simulink model "D53_LKAS"  (R2018b)
settings: Solver=ode3  StartTime=0.0  StopTime=10  FixedStep=0.01  RelTol=1e-3  EnableMultiTasking=on
model workspace (MAT data in the model file):
  MCOS : class17 (value not decoded)
  MCOS : class17 (value not decoded)
  MCOS : class17 (value not decoded)
  MCOS : class17 (value not decoded)
  MCOS : class17 (value not decoded)
  MCOS : class17 (value not decoded)
  MCOS : class17 (value not decoded)
  MCOS : class17 (value not decoded)
  MCOS : class17 (value not decoded)
  MCOS : class17 (value not decoded)
  MCOS : class17 (value not decoded)
  MCOS : class17 (value not decoded)
  MCOS : class17 (value not decoded)
  MCOS : class17 (value not decoded)
  MCOS : class17 (value not decoded)
  MCOS : class17 (value not decoded)
  MCOS : class17 (value not decoded)
  MCOS : class17 (value not decoded)
  MCOS : class17 (value not decoded)
  MCOS : class17 (value not decoded)
  MCOS : class17 (value not decoded)
  MCOS : class17 (value not decoded)
  MCOS : class17 (value not decoded)
  MCOS : class17 (value not decoded)
  MCOS : class17 (value not decoded)
  MCOS : class17 (value not decoded)
  MCOS : class17 (value not decoded)
  MCOS : class17 (value not decoded)
  MCOS : class17 (value not decoded)
  MCOS : class17 (value not decoded)
  MCOS : class17 (value not decoded)
  MCOS : class17 (value not decoded)
  MCOS : class17 (value not decoded)
  MCOS : class17 (value not decoded)
  MCOS : class17 (value not decoded)
  MCOS : class17 (value not decoded)
  MCOS : class17 (value not decoded)
  MCOS : class17 (value not decoded)
  MCOS : class17 (value not decoded)
  MCOS : class17 (value not decoded)
  MCOS : class17 (value not decoded)
  MCOS : class17 (value not decoded)
  MCOS : class17 (value not decoded)
  MCOS : class17 (value not decoded)
  MCOS : class17 (value not decoded)
  MCOS : class17 (value not decoded)
  MCOS : class17 (value not decoded)
  MCOS : class17 (value not decoded)
  MCOS : class17 (value not decoded)
  MCOS : class17 (value not decoded)
  MCOS : class17 (value not decoded)
  MCOS : class17 (value not decoded)
  MCOS : class17 (value not decoded)
  MCOS : class17 (value not decoded)
  MCOS : class17 (value not decoded)
  MCOS : class17 (value not decoded)
  MCOS : class17 (value not decoded)
  MCOS : class17 (value not decoded)
  MCOS : class17 (value not decoded)
  MCOS : class17 (value not decoded)
  MCOS : class17 (value not decoded)
  MCOS : class17 (value not decoded)
  MCOS : class17 (value not decoded)
  MCOS : class17 (value not decoded)
  MCOS : class17 (value not decoded)
  MCOS : class17 (value not decoded)
  MCOS : class17 (value not decoded)
  MCOS : class17 (value not decoded)
  MCOS : class17 (value not decoded)
  MCOS : class17 (value not decoded)
  MCOS : class17 (value not decoded)
  MCOS : class17 (value not decoded)
  MCOS : class17 (value not decoded)
  MCOS : class17 (value not decoded)
  MCOS : class17 (value not decoded)
  MCOS : class17 (value not decoded)
  MCOS : class17 (value not decoded)
  MCOS : class17 (value not decoded)
  MCOS : class17 (value not decoded)
  MCOS : class17 (value not decoded)
  MCOS : class17 (value not decoded)
  MCOS : class17 (value not decoded)
  MCOS : class17 (value not decoded)
  MCOS : class17 (value not decoded)
  MCOS : class17 (value not decoded)
  MCOS : class17 (value not decoded)
  MCOS : class17 (value not decoded)
  MCOS : class17 (value not decoded)
  MCOS : class17 (value not decoded)
values from neighbouring files (symbols this model uses):
  C = who    [Data_Process.m]
undefined symbols (not defined in the file or in its folder): LKA_CarWidth, LKA_SampleTime, LKA_StrRatio_C, LKA_Veh2CamL_C, LKA_Veh2CamW_C, LKA_WhlBaseL_C, LL_CompSWA_C, LL_CrvtPrvwT_C, LL_DesDvt_C, LL_DvtComp_C, LL_DvtPrvwT_C, LL_DvtSpdDet_vDvtSpdMin_C, LL_HdAgExT_C, LL_HdAgPrvwT_C, LL_LAccMax_C, LL_LAccRMax_C, LL_LDW_EarliestWarnLine_C, LL_LDW_LatestWarnLine_C, LL_LDWS_SUPPRESS_HEADING, LL_LFClb_TFC_DiffCtlBalance, LL_LFClb_TFC_DiffCtrlMaxSWA, LL_LFClb_TFC_DiffCtrlRatio, LL_LFClb_TFC_facmGainLutGain1_C, LL_LFClb_TFC_facmGainLutGain2_C, LL_LFClb_TFC_facmIntegRatio, LL_LFClb_TFC_facmKlat_C, LL_LFClb_TFC_FfCtlRatio_C, LL_LFClb_TFC_phiIntegCtlMaxSWA_C, LL_LFClb_TFC_tiKlatPrvwT_C, LL_LFClb_TFC_vGainLutVehSpdLwr_C, LL_LFClb_TFC_vGainLutVehSpdUpr_C, LL_LKA_EarliestWarnLine_C, LL_LKA_LatestWarnLine_C, LL_LKAExPrcs_ExitC0Dvt, LL_LKAExPrcs_ExitC0Swt, LL_LKAExPrcs_tiExitTime1, LL_LKAExPrcs_tiExitTime2, LL_LKAExPrcs_tiExitTime3, LL_LKAS_OUT_OF_CONTROL_LAT_VEL, LL_LKAS_OUT_OF_CONTROL_TTLC, LL_LKASWASyn_M0, LL_LKASWASyn_M1, LL_LKASWASyn_M2, LL_LKASWASyn_M3K, LL_LKASWASyn_SWAaddMax, LL_LKASWASyn_T2, LL_LKASWASyn_tiTrqSwaRtTime, LL_LKASWASyn_tiTrqSwaTime, LL_LKASWASyn_TrqMax, LL_LKASWASyn_TrqSwaAddSwt, LL_LKASWASyn_TrqSwaRateDiff, LL_LSpdCompT_C, LL_lStpLngth_C, LL_MAX_DELAY_EPSSTAR_TIME, LL_MAX_DRIVER_TORQUE_DISABLE, LL_MAX_DRIVER_TORQUE_ENABLE, LL_MAX_LANE_WIDTH_DISABLE, LL_MAX_LANE_WIDTH_ENABLE, LL_MAX_LAT_ACC_DISABLE, LL_MAX_LAT_ACC_ENABLE ... (+30)
libraries: simulink x134, canmsglib x52, dspstat3 x3, simulink_extras x1
(part 6 of 18)

== system D53_LKAS/SignalBusCreator/bsOriR0Info ==
  Bus Creator21 : BusCreator  Inputs=10
  CAN Pack : canmsglib/CAN Pack  CANdbFile=D:\LKAS\Documents\LKAS-Monitor.dbc  MsgList=Video_Lane_Right_B  MsgName=Video_Lane_Right_B  MsgIDType=Standard (11-bit identifier)  MsgIdentifier=1791  MsgLength=4  SignalInfo=Line_Width_5FF$17$7$2$2$1$0$1.000000e-02$0$0$1.270000e+00$#Me_Line_Changed_5FF$16$1$2$2$1$0$1$0$0$1$#TLC_5FF$8$8$2$2$1$0$1.000000e-02$0$0$2.550000e+00$#View_Range_5FF$0$8$2$2$1$0$5.000000e-01$0$0$1.275000e+02$#  NSignals=4  StartBits=str2num('[int32(17);int32(16);int32(8);int32(0)]')  SignalSizes=str2num('[int32(7);int32(1);int32(8);int32(8)]')  ByteOrders=str2num('[int32(2);int32(2);int32(2);int32(2)]')  DataTypes=str2num('[int32(2);int32(2);int32(2);int32(2)]')  MultiplexTypes=str2num('[int32(1);int32(1);int32(1);int32(1)]')  MultiplexValues=str2num('[double(0);double(0);double(0);double(0)]')  Factors=str2num('[double(1.000000e-02);double(1);double(1.000000e-02);double(5.000000e-01)]')  Offsets=str2num('[double(0);double(0);double(0);double(0)]')  Minimums=str2num('[double(0);double(0);double(0);double(0)]')  Maximums=str2num('[double(1.270000e+00);double(1);double(2.550000e+00);double(1.275000e+02)]')  Remote=off  ApplyMinMax=off  BusOutput=off
      settings: SourceProductName=Simulink Real-Time  SourceProductBaseCode=XP  DataFormat=CANdb specified signals
  CAN Pack1 : canmsglib/CAN Pack  CANdbFile=D:\LKAS\Documents\LKAS-Monitor.dbc  MsgList=Video_Lane_Right_A  MsgName=Video_Lane_Right_A  MsgIDType=Standard (11-bit identifier)  MsgIdentifier=1789  MsgLength=8  SignalInfo=C0_5FD$44$12$2$1$1$0$1.000000e-02$0$-2.048000e+01$2.047000e+01$#C1_5FD$50$10$2$1$1$0$9.765625e-04$0$-3.570000e-01$3.570000e-01$#C2_5FD$24$16$2$1$1$0$1.000000e-06$0$-3.276800e-02$3.276600e-02$#C3_5FD$8$16$2$1$1$0$4.000000e-09$0$-1.310720e-04$1.310680e-04$#Line_Type_5FD$59$3$2$2$1$0$1$0$0$7$#Quality_5FD$62$2$2$2$1$0$1$0$0$3$#  NSignals=6  StartBits=str2num('[int32(44);int32(50);int32(24);int32(8);int32(59);int32(62)]')  SignalSizes=str2num('[int32(12);int32(10);int32(16);int32(16);int32(3);int32(2)]')  ByteOrders=str2num('[int32(2);int32(2);int32(2);int32(2);int32(2);int32(2)]')  DataTypes=str2num('[int32(1);int32(1);int32(1);int32(1);int32(2);int32(2)]')  MultiplexTypes=str2num('[int32(1);int32(1);int32(1);int32(1);int32(1);int32(1)]')  MultiplexValues=str2num('[double(0);double(0);double(0);double(0);double(0);double(0)]')  Factors=str2num('[double(1.000000e-02);double(9.765625e-04);double(1.000000e-06);double(4.000000e-09);double(1);double(1)]')  Offsets=str2num('[double(0);double(0);double(0);double(0);double(0);double(0)]')  Minimums=str2num('[double(-2.048000e+01);double(-3.570000e-01);double(-3.276800e-02);double(-1.310720e-04);double(0);double(0)]')  Maximums=str2num('[double(2.047000e+01);double(3.570000e-01);double(3.276600e-02);double(1.310680e-04);double(7);double(3)]')  Remote=off  ApplyMinMax=off  BusOutput=off
      settings: SourceProductName=Simulink Real-Time  SourceProductBaseCode=XP  DataFormat=CANdb specified signals
  CAN Pack2 : canmsglib/CAN Pack  CANdbFile=D:\LKAS\Documents\D53-PSA1CAN.dbc  MsgList=ADAS_44B_PSA1  MsgName=ADAS_44B_PSA1  MsgIDType=Standard (11-bit identifier)  MsgIdentifier=1099  MsgLength=8  SignalInfo=C0_coefficient44B$44$12$2$1$1$0$1.000000e-02$0$-2.048000e+01$2.047000e+01$#C1_coefficient44B$50$10$2$1$1$0$9.800000e-04$0$-3.570000e-01$3.570000e-01$#C2_coefficient44B$24$16$2$1$1$0$1.000000e-06$0$-3.276800e-02$3.276600e-02$#C3_coefficient44B$8$16$2$1$1$0$4.000000e-09$0$-1.310000e-04$1.310700e-04$#Detected_line_type44B$59$3$2$2$1$0$1$0$0$7$#Message_counter44B$48$2$2$2$1$0$1$0$0$3$#Quality_of_the_detected_line44B$62$2$2$2$1$0$1$0$0$3$#  NSignals=7  StartBits=str2num('[int32(44);int32(50);int32(24);int32(8);int32(59);int32(48);int32(62)]')  SignalSizes=str2num('[int32(12);int32(10);int32(16);int32(16);int32(3);int32(2);int32(2)]')  ByteOrders=str2num('[int32(2);int32(2);int32(2);int32(2);int32(2);int32(2);int32(2)]')  DataTypes=str2num('[int32(1);int32(1);int32(1);int32(1);int32(2);int32(2);int32(2)]')  MultiplexTypes=str2num('[int32(1);int32(1);int32(1);int32(1);int32(1);int32(1);int32(1)]')  MultiplexValues=str2num('[double(0);double(0);double(0);double(0);double(0);double(0);double(0)]')  Factors=str2num('[double(1.000000e-02);double(9.800000e-04);double(1.000000e-06);double(4.000000e-09);double(1);double(1);double(1)]')  Offsets=str2num('[double(0);double(0);double(0);double(0);double(0);double(0);double(0)]')  Minimums=str2num('[double(-2.048000e+01);double(-3.570000e-01);double(-3.276800e-02);double(-1.310000e-04);double(0);double(0);double(0)]')  Maximums=str2num('[double(2.047000e+01);double(3.570000e-01);double(3.276600e-02);double(1.310700e-04);double(7);double(3);double(3)]')  Remote=off  ApplyMinMax=off  BusOutput=off
      settings: SourceProductName=Simulink Real-Time  SourceProductBaseCode=XP  DataFormat=CANdb specified signals
  CAN Receive (CANRX) : S-Function  FunctionName=CAN_Rec_P  Parameters=uint8(Module-1),uint32(ID),uint8(Frameformat-1),uint8(Newflag),uint8(FIFO),double(sampletime)  SFunctionDeploymentMode=off  EnableBusSupport=off  mask(CAN_receive){Module=CAN_2, ID=1533, Frameformat=Standard (11-bit identifier), Newflag=on, FIFO=off, sampletime=0.05}
      mask prompts: Module "CAN Port:"; ID "CAN Frame ID:"; Frameformat "CAN Frame Format:"; FIFO "Overflow flag"
      mask init:
      | maskdisplay = canrecicon(Module,ID,Frameformat,Newflag,FIFO);
      | set_param(gcb, 'MaskDisplay', maskdisplay);
      mask TypeOptions Module: CAN_0 | CAN_1 | CAN_2 | CAN_3
      mask TypeOptions Frameformat: Standard (11-bit identifier) | Extended (29-bit identifier)
      mask Display: color('blue');text(0.98,0.9,'MPC5675K','horizontalAlignment','right');color('black');text(0.5,0.6,'FlexCAN_2 Receive','horizontalAlignment','center');text(0.5,0.35,'Standard ID:1533','horizontalAlignment','center');port_label('output',1,'New_Flag');port_label('output',2,'CAN_Msg');
  CAN Receive (CANRX)1 : S-Function  FunctionName=CAN_Rec_P  Parameters=uint8(Module-1),uint32(ID),uint8(Frameformat-1),uint8(Newflag),uint8(FIFO),double(sampletime)  SFunctionDeploymentMode=off  EnableBusSupport=off  mask(CAN_receive){Module=CAN_2, ID=1535, Frameformat=Standard (11-bit identifier), Newflag=on, FIFO=off, sampletime=0.05}
      mask prompts: Module "CAN Port:"; ID "CAN Frame ID:"; Frameformat "CAN Frame Format:"; FIFO "Overflow flag"
      mask init:
      | maskdisplay = canrecicon(Module,ID,Frameformat,Newflag,FIFO);
      | set_param(gcb, 'MaskDisplay', maskdisplay);
      mask TypeOptions Module: CAN_0 | CAN_1 | CAN_2 | CAN_3
      mask TypeOptions Frameformat: Standard (11-bit identifier) | Extended (29-bit identifier)
      mask Display: color('blue');text(0.98,0.9,'MPC5675K','horizontalAlignment','right');color('black');text(0.5,0.6,'FlexCAN_2 Receive','horizontalAlignment','center');text(0.5,0.35,'Standard ID:1535','horizontalAlignment','center');port_label('output',1,'New_Flag');port_label('output',2,'CAN_Msg');
  CAN Send1 : S-Function  FunctionName=CAN_Send_P  Parameters=uint8(CAN_Port-1),uint8(CAN_Priority-1),uint8(S_overflow_flag),uint8(S_timestamp),double(sampletime)  SFunctionDeploymentMode=off  EnableBusSupport=off  mask{CAN_Port=CAN_1, CAN_Priority=3, S_overflow_flag=off, S_timestamp=off, sampletime=0.05}
      mask prompts: CAN_Port "CAN Port:"; CAN_Priority "Priority:"; S_overflow_flag "Send overflow flag"; S_timestamp "Send time stamp"
      mask init:
      | maskdisplay = cansendicon(CAN_Port,CAN_Priority,S_overflow_flag,S_timestamp);
      | set_param(gcb, 'MaskDisplay', maskdisplay);
      mask TypeOptions CAN_Port: CAN_0 | CAN_1 | CAN_2 | CAN_3
      mask TypeOptions CAN_Priority: 0 | 1 | 2 | 3 | 4 | 5 | 6 | 7
      mask Display: color('blue');text(0.98,0.9,'MPC5675K','horizontalAlignment','right');color('black');text(0.5,0.6,'FlexCAN_1 Send','horizontalAlignment','center');text(0.5,0.35,'Priority:3','horizontalAlignment','center');port_label('input',1,'CAN_Msg');
  CAN Send2 : S-Function  FunctionName=CAN_Send_P  Parameters=uint8(CAN_Port-1),uint8(CAN_Priority-1),uint8(S_overflow_flag),uint8(S_timestamp),double(sampletime)  SFunctionDeploymentMode=off  EnableBusSupport=off  mask{CAN_Port=CAN_0, CAN_Priority=3, S_overflow_flag=off, S_timestamp=off, sampletime=0.05}
      mask prompts: CAN_Port "CAN Port:"; CAN_Priority "Priority:"; S_overflow_flag "Send overflow flag"; S_timestamp "Send time stamp"
      mask init:
      | maskdisplay = cansendicon(CAN_Port,CAN_Priority,S_overflow_flag,S_timestamp);
      | set_param(gcb, 'MaskDisplay', maskdisplay);
      mask TypeOptions CAN_Port: CAN_0 | CAN_1 | CAN_2 | CAN_3
      mask TypeOptions CAN_Priority: 0 | 1 | 2 | 3 | 4 | 5 | 6 | 7
      mask Display: color('blue');text(0.98,0.9,'MPC5675K','horizontalAlignment','right');color('black');text(0.5,0.6,'FlexCAN_0 Send','horizontalAlignment','center');text(0.5,0.35,'Priority:3','horizontalAlignment','center');port_label('input',1,'CAN_Msg');
  CAN Send3 : S-Function  FunctionName=CAN_Send_P  Parameters=uint8(CAN_Port-1),uint8(CAN_Priority-1),uint8(S_overflow_flag),uint8(S_timestamp),double(sampletime)  SFunctionDeploymentMode=off  EnableBusSupport=off  mask{CAN_Port=CAN_0, CAN_Priority=3, S_overflow_flag=off, S_timestamp=off, sampletime=0.05}
      mask prompts: CAN_Port "CAN Port:"; CAN_Priority "Priority:"; S_overflow_flag "Send overflow flag"; S_timestamp "Send time stamp"
      mask init:
      | maskdisplay = cansendicon(CAN_Port,CAN_Priority,S_overflow_flag,S_timestamp);
      | set_param(gcb, 'MaskDisplay', maskdisplay);
      mask TypeOptions CAN_Port: CAN_0 | CAN_1 | CAN_2 | CAN_3
      mask TypeOptions CAN_Priority: 0 | 1 | 2 | 3 | 4 | 5 | 6 | 7
      mask Display: color('blue');text(0.98,0.9,'MPC5675K','horizontalAlignment','right');color('black');text(0.5,0.6,'FlexCAN_0 Send','horizontalAlignment','center');text(0.5,0.35,'Priority:3','horizontalAlignment','center');port_label('input',1,'CAN_Msg');
  CAN Unpack1 : canmsglib/CAN Unpack  CANdbFile=D:\Work\02_LKA\LKAS\Documents\D53-SensorCAN.dbc  MsgList=Video_Lane_Right_B  MsgName=Video_Lane_Right_B  MsgIDType=Standard (11-bit identifier)  MsgIdentifier=1535  MsgLength=4  SignalInfo=Line_Width_5FF$17$7$2$2$1$0$1.000000e-02$0$0$1.270000e+00$#Me_Line_Changed_5FF$16$1$2$2$1$0$1$0$0$1$#TLC_5FF$8$8$2$2$1$0$1.000000e-02$0$0$2.550000e+00$#View_Range_5FF$0$8$2$2$1$0$5.000000e-01$0$0$1.275000e+02$#  NSignals=4  IDPort=off  TimestampPort=off  ErrorPort=off  RemotePort=off  LengthPort=off  StatusPort=off  StartBits=str2num('[int32(17);int32(16);int32(8);int32(0)]')  SignalSizes=str2num('[int32(7);int32(1);int32(8);int32(8)]')  ByteOrders=str2num('[int32(2);int32(2);int32(2);int32(2)]')  DataTypes=str2num('[int32(2);int32(2);int32(2);int32(2)]')  MultiplexTypes=str2num('[int32(1);int32(1);int32(1);int32(1)]')  MultiplexValues=str2num('[double(0);double(0);double(0);double(0)]')  Factors=str2num('[double(1.000000e-02);double(1);double(1.000000e-02);double(5.000000e-01)]')  Offsets=str2num('[double(0);double(0);double(0);double(0)]')  Minimums=str2num('[double(0);double(0);double(0);double(0)]')  Maximums=str2num('[double(1.270000e+00);double(1);double(2.550000e+00);double(1.275000e+02)]')  ApplyMinMax=off
      settings: SourceProductName=Simulink Real-Time  SourceProductBaseCode=XP  DataFormat=CANdb specified signals
  CAN Unpack14 : canmsglib/CAN Unpack  CANdbFile=D:\Work\02_LKA\LKAS\Documents\D53-SensorCAN.dbc  MsgList=Video_Lane_Right_A  MsgName=Video_Lane_Right_A  MsgIDType=Standard (11-bit identifier)  MsgIdentifier=1533  MsgLength=8  SignalInfo=C0_5FD$44$12$2$1$1$0$1.000000e-02$0$-2.048000e+01$2.047000e+01$#C1_5FD$50$10$2$1$1$0$9.765625e-04$0$-3.570000e-01$3.570000e-01$#C2_5FD$24$16$2$1$1$0$1.000000e-06$0$-3.276800e-02$3.276600e-02$#C3_5FD$8$16$2$1$1$0$4.000000e-09$0$-1.310720e-04$1.310680e-04$#Line_Type_5FD$59$3$2$2$1$0$1$0$0$7$#Quality_5FD$62$2$2$2$1$0$1$0$0$3$#  NSignals=6  IDPort=off  TimestampPort=off  ErrorPort=off  RemotePort=off  LengthPort=off  StatusPort=off  StartBits=str2num('[int32(44);int32(50);int32(24);int32(8);int32(59);int32(62)]')  SignalSizes=str2num('[int32(12);int32(10);int32(16);int32(16);int32(3);int32(2)]')  ByteOrders=str2num('[int32(2);int32(2);int32(2);int32(2);int32(2);int32(2)]')  DataTypes=str2num('[int32(1);int32(1);int32(1);int32(1);int32(2);int32(2)]')  MultiplexTypes=str2num('[int32(1);int32(1);int32(1);int32(1);int32(1);int32(1)]')  MultiplexValues=str2num('[double(0);double(0);double(0);double(0);double(0);double(0)]')  Factors=str2num('[double(1.000000e-02);double(9.765625e-04);double(1.000000e-06);double(4.000000e-09);double(1);double(1)]')  Offsets=str2num('[double(0);double(0);double(0);double(0);double(0);double(0)]')  Minimums=str2num('[double(-2.048000e+01);double(-3.570000e-01);double(-3.276800e-02);double(-1.310720e-04);double(0);double(0)]')  Maximums=str2num('[double(2.047000e+01);double(3.570000e-01);double(3.276600e-02);double(1.310680e-04);double(7);double(3)]')  ApplyMinMax=off
      settings: SourceProductName=Simulink Real-Time  SourceProductBaseCode=XP  DataFormat=CANdb specified signals
  Data Type Conversion{1..4,6..7,10} (7 alike) : DataTypeConversion  OutDataTypeStr=single
  Data Type Conversion5 : DataTypeConversion  OutDataTypeStr=uint8
  Data Type Conversion8 : DataTypeConversion  OutDataTypeStr=uint8
  Data Type Conversion9 : DataTypeConversion  OutDataTypeStr=uint8
  Ground : Ground
  Rate Transition{1..10} (10 alike) : RateTransition  Deterministic=off  OutPortSampleTime=0.01
  Rate Transition{11..27} (17 alike) : RateTransition  Deterministic=off  OutPortSampleTime=0.05
  bsOriR0Info : Outport
  wires:
  Data Type Conversion4/1 -> Rate Transition11/1, Rate Transition18/1, Bus Creator21/4  "O_R0_C0"
  CAN Unpack1/4 -> Rate Transition1/1
  Data Type Conversion1/1 -> Rate Transition12/1, Rate Transition19/1, Bus Creator21/3  "O_R0_C1"
  Data Type Conversion7/1 -> Rate Transition24/1, Bus Creator21/9  "O_R0_W"
  Data Type Conversion10/1 -> Rate Transition26/1, Bus Creator21/8  "O_R0_TLC"
  CAN Unpack1/2 -> Rate Transition3/1
  Data Type Conversion9/1 -> Rate Transition25/1, Bus Creator21/10  "O_R0_LC"
  Data Type Conversion6/1 -> Rate Transition27/1, Bus Creator21/7  "O_R0_VR"
  CAN Unpack14/1 -> Rate Transition10/1
  Data Type Conversion2/1 -> Rate Transition20/1, Rate Transition13/1, Bus Creator21/2  "O_R0_C2"
  CAN Unpack14/3 -> Rate Transition8/1
  CAN Unpack1/3 -> Rate Transition2/1
  Data Type Conversion8/1 -> Rate Transition22/1, Rate Transition15/1, Bus Creator21/6  "O_R0_Type"
  Data Type Conversion3/1 -> Rate Transition21/1, Rate Transition14/1, Bus Creator21/1  "O_R0_C3"
  CAN Unpack14/6 -> Rate Transition5/1
  CAN Unpack14/2 -> Rate Transition9/1
  CAN Unpack14/4 -> Rate Transition7/1
  CAN Unpack14/5 -> Rate Transition6/1
  Data Type Conversion5/1 -> Rate Transition23/1, Rate Transition16/1, Bus Creator21/5  "O_R0_Q"
  CAN Unpack1/1 -> Rate Transition4/1
  Bus Creator21/1 -> bsOriR0Info/1  "bsOriR0Info"
  Rate Transition1/1 -> Data Type Conversion6/1
  Rate Transition2/1 -> Data Type Conversion10/1
  Rate Transition3/1 -> Data Type Conversion9/1
  Rate Transition4/1 -> Data Type Conversion7/1
  Rate Transition5/1 -> Data Type Conversion5/1
  Rate Transition6/1 -> Data Type Conversion8/1
  Rate Transition7/1 -> Data Type Conversion3/1
  Rate Transition9/1 -> Data Type Conversion1/1
  Rate Transition8/1 -> Data Type Conversion2/1
  Rate Transition10/1 -> Data Type Conversion4/1
  CAN Pack/1 -> CAN Send3/1
  CAN Pack1/1 -> CAN Send2/1
  Ground/1 -> Rate Transition17/1
  CAN Pack2/1 -> CAN Send1/1
  Rate Transition11/1 -> CAN Pack2/1
  Rate Transition12/1 -> CAN Pack2/2
  Rate Transition13/1 -> CAN Pack2/3
  Rate Transition14/1 -> CAN Pack2/4
  Rate Transition15/1 -> CAN Pack2/5
  Rate Transition16/1 -> CAN Pack2/7
  Rate Transition17/1 -> CAN Pack2/6
  Rate Transition18/1 -> CAN Pack1/1
  Rate Transition19/1 -> CAN Pack1/2
  Rate Transition20/1 -> CAN Pack1/3
  Rate Transition21/1 -> CAN Pack1/4
  Rate Transition22/1 -> CAN Pack1/5
  Rate Transition23/1 -> CAN Pack1/6
  Rate Transition24/1 -> CAN Pack/1
  Rate Transition25/1 -> CAN Pack/2
  Rate Transition26/1 -> CAN Pack/3
  Rate Transition27/1 -> CAN Pack/4
  CAN Receive (CANRX)/2 -> CAN Unpack14/1
  CAN Receive (CANRX)1/2 -> CAN Unpack1/1

== system D53_LKAS/SignalBusCreator/bsOriR1Info ==
  Bus Creator22 : BusCreator  Inputs=10
  CAN Receive (CANRX) : S-Function  FunctionName=CAN_Rec_P  Parameters=uint8(Module-1),uint32(ID),uint8(Frameformat-1),uint8(Newflag),uint8(FIFO),double(sampletime)  SFunctionDeploymentMode=off  EnableBusSupport=off  mask(CAN_receive){Module=CAN_2, ID=1534, Frameformat=Standard (11-bit identifier), Newflag=on, FIFO=off, sampletime=0.05}
      mask prompts: Module "CAN Port:"; ID "CAN Frame ID:"; Frameformat "CAN Frame Format:"; FIFO "Overflow flag"
      mask init:
      | maskdisplay = canrecicon(Module,ID,Frameformat,Newflag,FIFO);
      | set_param(gcb, 'MaskDisplay', maskdisplay);
      mask TypeOptions Module: CAN_0 | CAN_1 | CAN_2 | CAN_3
      mask TypeOptions Frameformat: Standard (11-bit identifier) | Extended (29-bit identifier)
      mask Display: color('blue');text(0.98,0.9,'MPC5675K','horizontalAlignment','right');color('black');text(0.5,0.6,'FlexCAN_2 Receive','horizontalAlignment','center');text(0.5,0.35,'Standard ID:1534','horizontalAlignment','center');port_label('output',1,'New_Flag');port_label('output',2,'CAN_Msg');
  CAN Receive (CANRX)1 : S-Function  FunctionName=CAN_Rec_P  Parameters=uint8(Module-1),uint32(ID),uint8(Frameformat-1),uint8(Newflag),uint8(FIFO),double(sampletime)  SFunctionDeploymentMode=off  EnableBusSupport=off  mask(CAN_receive){Module=CAN_2, ID=1524, Frameformat=Standard (11-bit identifier), Newflag=on, FIFO=off, sampletime=0.05}
      mask prompts: Module "CAN Port:"; ID "CAN Frame ID:"; Frameformat "CAN Frame Format:"; FIFO "Overflow flag"
      mask init:
      | maskdisplay = canrecicon(Module,ID,Frameformat,Newflag,FIFO);
      | set_param(gcb, 'MaskDisplay', maskdisplay);
      mask TypeOptions Module: CAN_0 | CAN_1 | CAN_2 | CAN_3
      mask TypeOptions Frameformat: Standard (11-bit identifier) | Extended (29-bit identifier)
      mask Display: color('blue');text(0.98,0.9,'MPC5675K','horizontalAlignment','right');color('black');text(0.5,0.6,'FlexCAN_2 Receive','horizontalAlignment','center');text(0.5,0.35,'Standard ID:1524','horizontalAlignment','center');port_label('output',1,'New_Flag');port_label('output',2,'CAN_Msg');
  CAN Unpack1 : canmsglib/CAN Unpack  CANdbFile=D:\Work\02_LKA\LKAS\Documents\D53-SensorCAN.dbc  MsgList=Video_Lane_Next_Right_B  MsgName=Video_Lane_Next_Right_B  MsgIDType=Standard (11-bit identifier)  MsgIdentifier=1524  MsgLength=4  SignalInfo=Line_Width_5F4$17$7$2$2$1$0$1.000000e-02$0$0$1.270000e+00$#Me_Line_Changed_5F4$16$1$2$2$1$0$1$0$0$1$#TLC_5F4$8$8$2$2$1$0$1.000000e-02$0$0$2.550000e+00$#View_Range_5F4$0$8$2$2$1$0$5.000000e-01$0$0$1.275000e+02$#  NSignals=4  IDPort=off  TimestampPort=off  ErrorPort=off  RemotePort=off  LengthPort=off  StatusPort=off  StartBits=str2num('[int32(17);int32(16);int32(8);int32(0)]')  SignalSizes=str2num('[int32(7);int32(1);int32(8);int32(8)]')  ByteOrders=str2num('[int32(2);int32(2);int32(2);int32(2)]')  DataTypes=str2num('[int32(2);int32(2);int32(2);int32(2)]')  MultiplexTypes=str2num('[int32(1);int32(1);int32(1);int32(1)]')  MultiplexValues=str2num('[double(0);double(0);double(0);double(0)]')  Factors=str2num('[double(1.000000e-02);double(1);double(1.000000e-02);double(5.000000e-01)]')  Offsets=str2num('[double(0);double(0);double(0);double(0)]')  Minimums=str2num('[double(0);double(0);double(0);double(0)]')  Maximums=str2num('[double(1.270000e+00);double(1);double(2.550000e+00);double(1.275000e+02)]')  ApplyMinMax=off
      settings: SourceProductName=Simulink Real-Time  SourceProductBaseCode=XP  DataFormat=CANdb specified signals
  CAN Unpack13 : canmsglib/CAN Unpack  CANdbFile=D:\Work\02_LKA\LKAS\Documents\D53-SensorCAN.dbc  MsgList=Video_Lane_Next_Right_A  MsgName=Video_Lane_Next_Right_A  MsgIDType=Standard (11-bit identifier)  MsgIdentifier=1534  MsgLength=8  SignalInfo=C0_5FE$44$12$2$1$1$0$1.000000e-02$0$-2.048000e+01$2.047000e+01$#C1_5FE$50$10$2$1$1$0$9.765625e-04$0$-3.570000e-01$3.570000e-01$#C2_5FE$24$16$2$1$1$0$1.000000e-06$0$-3.276800e-02$3.276600e-02$#C3_5FE$8$16$2$1$1$0$4.000000e-09$0$-1.310720e-04$1.310680e-04$#Line_Type_5FE$59$3$2$2$1$0$1$0$0$7$#Quality_5FE$62$2$2$2$1$0$1$0$0$3$#  NSignals=6  IDPort=off  TimestampPort=off  ErrorPort=off  RemotePort=off  LengthPort=off  StatusPort=off  StartBits=str2num('[int32(44);int32(50);int32(24);int32(8);int32(59);int32(62)]')  SignalSizes=str2num('[int32(12);int32(10);int32(16);int32(16);int32(3);int32(2)]')  ByteOrders=str2num('[int32(2);int32(2);int32(2);int32(2);int32(2);int32(2)]')  DataTypes=str2num('[int32(1);int32(1);int32(1);int32(1);int32(2);int32(2)]')  MultiplexTypes=str2num('[int32(1);int32(1);int32(1);int32(1);int32(1);int32(1)]')  MultiplexValues=str2num('[double(0);double(0);double(0);double(0);double(0);double(0)]')  Factors=str2num('[double(1.000000e-02);double(9.765625e-04);double(1.000000e-06);double(4.000000e-09);double(1);double(1)]')  Offsets=str2num('[double(0);double(0);double(0);double(0);double(0);double(0)]')  Minimums=str2num('[double(-2.048000e+01);double(-3.570000e-01);double(-3.276800e-02);double(-1.310720e-04);double(0);double(0)]')  Maximums=str2num('[double(2.047000e+01);double(3.570000e-01);double(3.276600e-02);double(1.310680e-04);double(7);double(3)]')  ApplyMinMax=off
      settings: SourceProductName=Simulink Real-Time  SourceProductBaseCode=XP  DataFormat=CANdb specified signals
  Data Type Conversion{,6..8,10..11,14} (7 alike) : DataTypeConversion  OutDataTypeStr=single
  Data Type Conversion12 : DataTypeConversion  OutDataTypeStr=uint8
  Data Type Conversion13 : DataTypeConversion  OutDataTypeStr=uint8
  Data Type Conversion9 : DataTypeConversion  OutDataTypeStr=uint8
  Rate Transition{1..10} (10 alike) : RateTransition  Deterministic=off  OutPortSampleTime=0.01
  bsOriR1Info : Outport
  wires:
  Data Type Conversion6/1 -> Bus Creator22/3  "O_R1_C1"
  Data Type Conversion11/1 -> Bus Creator22/9  "O_R1_W"
  Data Type Conversion14/1 -> Bus Creator22/8  "O_R1_TLC"
  Data Type Conversion/1 -> Bus Creator22/4  "O_R1_C0"
  Data Type Conversion7/1 -> Bus Creator22/2  "O_R1_C2"
  Data Type Conversion9/1 -> Bus Creator22/5  "O_R1_Q"
  Data Type Conversion13/1 -> Bus Creator22/10  "O_R1_LC"
  Data Type Conversion8/1 -> Bus Creator22/1  "O_R1_C3"
  CAN Unpack13/2 -> Rate Transition2/1
  CAN Unpack13/3 -> Rate Transition3/1
  Data Type Conversion12/1 -> Bus Creator22/6  "O_R1_Type"
  Data Type Conversion10/1 -> Bus Creator22/7  "O_R1_VR"
  CAN Unpack13/1 -> Rate Transition1/1
  CAN Unpack1/4 -> Rate Transition10/1
  CAN Unpack1/3 -> Rate Transition9/1
  CAN Unpack13/5 -> Rate Transition5/1
  CAN Unpack13/6 -> Rate Transition6/1
  CAN Unpack1/2 -> Rate Transition8/1
  CAN Unpack1/1 -> Rate Transition7/1
  CAN Unpack13/4 -> Rate Transition4/1
  Bus Creator22/1 -> bsOriR1Info/1  "bsOriR1Info"
  Rate Transition1/1 -> Data Type Conversion/1
  Rate Transition2/1 -> Data Type Conversion6/1
  Rate Transition3/1 -> Data Type Conversion7/1
  Rate Transition4/1 -> Data Type Conversion8/1
  Rate Transition5/1 -> Data Type Conversion12/1
  Rate Transition6/1 -> Data Type Conversion9/1
  Rate Transition7/1 -> Data Type Conversion11/1
  Rate Transition8/1 -> Data Type Conversion13/1
  Rate Transition9/1 -> Data Type Conversion14/1
  Rate Transition10/1 -> Data Type Conversion10/1
  CAN Receive (CANRX)/2 -> CAN Unpack13/1
  CAN Receive (CANRX)1/2 -> CAN Unpack1/1

== system D53_LKAS/SignalBusCreator/bsPTState ==
  Bus Creator4 : BusCreator  Inputs=2
  CAN Pack : canmsglib/CAN Pack  CANdbFile=D:\LKAS\Documents\LKAS-Monitor.dbc  MsgList=GW_349_PSA1  MsgName=GW_349_PSA1  MsgIDType=Standard (11-bit identifier)  MsgIdentifier=840  MsgLength=8  SignalInfo=TCU_Gear_lever_position$24$4$2$2$1$0$1$0$-Inf$Inf$#  NSignals=1  StartBits=str2num('[int32(24)]')  SignalSizes=str2num('[int32(4)]')  ByteOrders=str2num('[int32(2)]')  DataTypes=str2num('[int32(2)]')  MultiplexTypes=str2num('[int32(1)]')  MultiplexValues=str2num('[double(0)]')  Factors=str2num('[double(1)]')  Offsets=str2num('[double(0)]')  Minimums=str2num('[double(-Inf)]')  Maximums=str2num('[double(Inf)]')  Remote=off  ApplyMinMax=off  BusOutput=off
      settings: SourceProductName=Simulink Real-Time  SourceProductBaseCode=XP  DataFormat=CANdb specified signals
  CAN Send1 : S-Function  FunctionName=CAN_Send_P  Parameters=uint8(CAN_Port-1),uint8(CAN_Priority-1),uint8(S_overflow_flag),uint8(S_timestamp),double(sampletime)  SFunctionDeploymentMode=off  EnableBusSupport=off  mask{CAN_Port=CAN_0, CAN_Priority=3, S_overflow_flag=off, S_timestamp=off, sampletime=0.1}
      mask prompts: CAN_Port "CAN Port:"; CAN_Priority "Priority:"; S_overflow_flag "Send overflow flag"; S_timestamp "Send time stamp"
      mask init:
      | maskdisplay = cansendicon(CAN_Port,CAN_Priority,S_overflow_flag,S_timestamp);
      | set_param(gcb, 'MaskDisplay', maskdisplay);
      mask TypeOptions CAN_Port: CAN_0 | CAN_1 | CAN_2 | CAN_3
      mask TypeOptions CAN_Priority: 0 | 1 | 2 | 3 | 4 | 5 | 6 | 7
      mask Display: color('blue');text(0.98,0.9,'MPC5675K','horizontalAlignment','right');color('black');text(0.5,0.6,'FlexCAN_0 Send','horizontalAlignment','center');text(0.5,0.35,'Priority:3','horizontalAlignment','center');port_label('input',1,'CAN_Msg');
  CAN Unpack1 : canmsglib/CAN Unpack  CANdbFile=D:\Work\02_LKA\LKAS\Documents\D53-PSA1CAN.dbc  MsgList=GW_228_PSA1  MsgName=GW_228_PSA1  MsgIDType=Standard (11-bit identifier)  MsgIdentifier=552  MsgLength=8  SignalInfo=EMS_Acceleration_pedal_position$16$8$2$2$1$0$5.000000e-01$0$0$100$#  NSignals=1  IDPort=off  TimestampPort=off  ErrorPort=off  RemotePort=off  LengthPort=off  StatusPort=off  StartBits=str2num('[int32(16)]')  SignalSizes=str2num('[int32(8)]')  ByteOrders=str2num('[int32(2)]')  DataTypes=str2num('[int32(2)]')  MultiplexTypes=str2num('[int32(1)]')  MultiplexValues=str2num('[double(0)]')  Factors=str2num('[double(5.000000e-01)]')  Offsets=str2num('[double(0)]')  Minimums=str2num('[double(0)]')  Maximums=str2num('[double(100)]')  ApplyMinMax=off
      settings: SourceProductName=Simulink Real-Time  SourceProductBaseCode=XP  DataFormat=CANdb specified signals
  CAN Unpack6 : canmsglib/CAN Unpack  CANdbFile=D:\Work\02_LKA\LKAS\Documents\D53-PSA1CAN.dbc  MsgList=GW_349_PSA1  MsgName=GW_349_PSA1  MsgIDType=Standard (11-bit identifier)  MsgIdentifier=841  MsgLength=8  SignalInfo=BV_dynamic_frame_checksum$52$4$2$2$1$0$1$0$-Inf$Inf$#TCU_AGB_Target_position$28$4$2$2$1$0$1$0$-Inf$Inf$#TCU_Gear_lever_position$24$4$2$2$1$0$1$0$-Inf$Inf$#bits_Compute_for_Gear_Box$48$4$2$2$1$0$1$0$0$15$#  NSignals=4  IDPort=off  TimestampPort=off  ErrorPort=off  RemotePort=off  LengthPort=off  StatusPort=off  StartBits=str2num('[int32(52);int32(28);int32(24);int32(48)]')  SignalSizes=str2num('[int32(4);int32(4);int32(4);int32(4)]')  ByteOrders=str2num('[int32(2);int32(2);int32(2);int32(2)]')  DataTypes=str2num('[int32(2);int32(2);int32(2);int32(2)]')  MultiplexTypes=str2num('[int32(1);int32(1);int32(1);int32(1)]')  MultiplexValues=str2num('[double(0);double(0);double(0);double(0)]')  Factors=str2num('[double(1);double(1);double(1);double(1)]')  Offsets=str2num('[double(0);double(0);double(0);double(0)]')  Minimums=str2num('[double(-Inf);double(-Inf);double(-Inf);double(0)]')  Maximums=str2num('[double(Inf);double(Inf);double(Inf);double(15)]')  ApplyMinMax=off
      settings: SourceProductName=Simulink Real-Time  SourceProductBaseCode=XP  DataFormat=CANdb specified signals
  CAN_Receive1 : S-Function  FunctionName=CAN_Rec_P  Parameters=uint8(Module-1),uint32(ID),uint8(Frameformat-1),uint8(Newflag),uint8(FIFO),double(sampletime)  SFunctionDeploymentMode=off  EnableBusSupport=off  mask(CAN_receive){Module=CAN_1, ID=552, Frameformat=Standard (11-bit identifier), Newflag=on, FIFO=off, sampletime=0.01}
      mask prompts: Module "CAN Port:"; ID "CAN Frame ID:"; Frameformat "CAN Frame Format:"; FIFO "Overflow flag"
      mask init:
      | maskdisplay = canrecicon(Module,ID,Frameformat,Newflag,FIFO);
      | set_param(gcb, 'MaskDisplay', maskdisplay);
      mask TypeOptions Module: CAN_0 | CAN_1 | CAN_2 | CAN_3
      mask TypeOptions Frameformat: Standard (11-bit identifier) | Extended (29-bit identifier)
      mask Display: color('blue');text(0.98,0.9,'MPC5675K','horizontalAlignment','right');color('black');text(0.5,0.6,'FlexCAN_1 Receive','horizontalAlignment','center');text(0.5,0.35,'Standard ID:552','horizontalAlignment','center');port_label('output',1,'New_Flag');port_label('output',2,'CAN_Msg');
  CAN_Receive6 : S-Function  FunctionName=CAN_Rec_P  Parameters=uint8(Module-1),uint32(ID),uint8(Frameformat-1),uint8(Newflag),uint8(FIFO),double(sampletime)  SFunctionDeploymentMode=off  EnableBusSupport=off  mask(CAN_receive){Module=CAN_1, ID=841, Frameformat=Standard (11-bit identifier), Newflag=on, FIFO=off, sampletime=0.01}
      mask prompts: Module "CAN Port:"; ID "CAN Frame ID:"; Frameformat "CAN Frame Format:"; FIFO "Overflow flag"
      mask init:
      | maskdisplay = canrecicon(Module,ID,Frameformat,Newflag,FIFO);
      | set_param(gcb, 'MaskDisplay', maskdisplay);
      mask TypeOptions Module: CAN_0 | CAN_1 | CAN_2 | CAN_3
      mask TypeOptions Frameformat: Standard (11-bit identifier) | Extended (29-bit identifier)
      mask Display: color('blue');text(0.98,0.9,'MPC5675K','horizontalAlignment','right');color('black');text(0.5,0.6,'FlexCAN_1 Receive','horizontalAlignment','center');text(0.5,0.35,'Standard ID:841','horizontalAlignment','center');port_label('output',1,'New_Flag');port_label('output',2,'CAN_Msg');
  Data Type Conversion1 : DataTypeConversion  OutDataTypeStr=uint8
  Data Type Conversion7 : DataTypeConversion  OutDataTypeStr=uint8
  Rate Transition1 : RateTransition  OutPortSampleTime=0.01
  Rate Transition{2..5} (4 alike) : RateTransition  Deterministic=off  OutPortSampleTime=0.01
  Rate Transition6 : RateTransition  Deterministic=off  OutPortSampleTime=0.1
  Terminator : Terminator
  Terminator1 : Terminator
  Terminator2 : Terminator
  bsPTState : Outport
  wires:
  CAN Unpack6/3 -> Rate Transition3/1
  Bus Creator4/1 -> bsPTState/1  "bsPTState"
  CAN Unpack6/1 -> Rate Transition2/1
  Data Type Conversion7/1 -> Rate Transition6/1, Bus Creator4/2  "TCU_ActualGear"
  CAN Unpack6/4 -> Rate Transition5/1
  CAN Unpack1/1 -> Rate Transition1/1
  Rate Transition1/1 -> Data Type Conversion1/1
  Data Type Conversion1/1 -> Bus Creator4/1  "AccPedal_Pos"
  CAN Unpack6/2 -> Rate Transition4/1
  Rate Transition3/1 -> Data Type Conversion7/1
  CAN Pack/1 -> CAN Send1/1
  Rate Transition2/1 -> Terminator/1
  Rate Transition4/1 -> Terminator2/1
  Rate Transition5/1 -> Terminator1/1
  Rate Transition6/1 -> CAN Pack/1
  CAN_Receive6/2 -> CAN Unpack6/1
  CAN_Receive1/2 -> CAN Unpack1/1

== system D53_LKAS/SignalBusCreator/bsSWAInfo ==
  Bus Creator3 : BusCreator  Inputs=4
  CAN Pack : canmsglib/CAN Pack  CANdbFile=D:\LKAS\Documents\LKAS-Monitor.dbc  MsgList=EPS_305_PSA1  MsgName=EPS_305_PSA1  MsgIDType=Standard (11-bit identifier)  MsgIdentifier=772  MsgLength=7  SignalInfo=Steering_wheel_angle$8$16$2$1$1$0$1.000000e-01$0$-780$780$#Steering_wheel_rotation_speed$16$8$2$2$1$0$4$0$0$1016$#Steering_wheel_sensor_direction$31$1$2$2$1$0$1$0$-Inf$Inf$#  NSignals=3  StartBits=str2num('[int32(8);int32(16);int32(31)]')  SignalSizes=str2num('[int32(16);int32(8);int32(1)]')  ByteOrders=str2num('[int32(2);int32(2);int32(2)]')  DataTypes=str2num('[int32(1);int32(2);int32(2)]')  MultiplexTypes=str2num('[int32(1);int32(1);int32(1)]')  MultiplexValues=str2num('[double(0);double(0);double(0)]')  Factors=str2num('[double(1.000000e-01);double(4);double(1)]')  Offsets=str2num('[double(0);double(0);double(0)]')  Minimums=str2num('[double(-780);double(0);double(-Inf)]')  Maximums=str2num('[double(780);double(1016);double(Inf)]')  Remote=off  ApplyMinMax=off  BusOutput=off
      settings: SourceProductName=Simulink Real-Time  SourceProductBaseCode=XP  DataFormat=CANdb specified signals
  CAN Recv (CANRx]) : S-Function  FunctionName=CAN_Rec_P  Parameters=uint8(Module-1),uint32(ID),uint8(Frameformat-1),uint8(Newflag),uint8(FIFO),double(sampletime)  SFunctionDeploymentMode=off  EnableBusSupport=off  mask(CAN_receive){Module=CAN_1, ID=773, Frameformat=Standard (11-bit identifier), Newflag=on, FIFO=off, sampletime=0.01}
      mask prompts: Module "CAN Port:"; ID "CAN Frame ID:"; Frameformat "CAN Frame Format:"; FIFO "Overflow flag"
      mask init:
      | maskdisplay = canrecicon(Module,ID,Frameformat,Newflag,FIFO);
      | set_param(gcb, 'MaskDisplay', maskdisplay);
      mask TypeOptions Module: CAN_0 | CAN_1 | CAN_2 | CAN_3
      mask TypeOptions Frameformat: Standard (11-bit identifier) | Extended (29-bit identifier)
      mask Display: color('blue');text(0.98,0.9,'MPC5675K','horizontalAlignment','right');color('black');text(0.5,0.6,'FlexCAN_1 Receive','horizontalAlignment','center');text(0.5,0.35,'Standard ID:773','horizontalAlignment','center');port_label('output',1,'New_Flag');port_label('output',2,'CAN_Msg');
  CAN Send2 : S-Function  FunctionName=CAN_Send_P  Parameters=uint8(CAN_Port-1),uint8(CAN_Priority-1),uint8(S_overflow_flag),uint8(S_timestamp),double(sampletime)  SFunctionDeploymentMode=off  EnableBusSupport=off  mask{CAN_Port=CAN_0, CAN_Priority=3, S_overflow_flag=off, S_timestamp=off, sampletime=0.1}
      mask prompts: CAN_Port "CAN Port:"; CAN_Priority "Priority:"; S_overflow_flag "Send overflow flag"; S_timestamp "Send time stamp"
      mask init:
      | maskdisplay = cansendicon(CAN_Port,CAN_Priority,S_overflow_flag,S_timestamp);
      | set_param(gcb, 'MaskDisplay', maskdisplay);
      mask TypeOptions CAN_Port: CAN_0 | CAN_1 | CAN_2 | CAN_3
      mask TypeOptions CAN_Priority: 0 | 1 | 2 | 3 | 4 | 5 | 6 | 7
      mask Display: color('blue');text(0.98,0.9,'MPC5675K','horizontalAlignment','right');color('black');text(0.5,0.6,'FlexCAN_0 Send','horizontalAlignment','center');text(0.5,0.35,'Priority:3','horizontalAlignment','center');port_label('input',1,'CAN_Msg');
  CAN Unpack1 : canmsglib/CAN Unpack  CANdbFile=D:\Work\02_LKA\LKAS\Documents\D53-PSA1CAN.dbc  MsgList=EPS_305_PSA1  MsgName=EPS_305_PSA1  MsgIDType=Standard (11-bit identifier)  MsgIdentifier=773  MsgLength=7  SignalInfo=Absolute_Steering_Wheel_angle$54$1$2$2$1$0$1$0$-Inf$Inf$#Initialization_steering_angle$55$1$2$2$1$0$1$0$-Inf$Inf$#Internal_SWS_status$24$1$2$2$1$0$1$0$-Inf$Inf$#SWS_calibration$25$1$2$2$1$0$1$0$-Inf$Inf$#SWS_checksum$36$4$2$2$1$0$1$0$-Inf$Inf$#SWS_fault_code$27$4$2$2$1$0$1$0$-Inf$Inf$#SWS_trim$26$1$2$2$1$0$1$0$-Inf$Inf$#Steering_wheel_angle$8$16$2$1$1$0$1.000000e-01$0$-780$780$#Steering_wheel_rotation_speed$16$8$2$2$1$0$4$0$0$1016$#Steering_wheel_sensor_direction$31$1$2$2$1$0$1$0$-Inf$Inf$#bits_Compute_counter_for_SWS$32$4$2$2$1$0$1$0$0$15$#indication_of_steering_wheel$52$2$2$2$1$0$1$0$-Inf$Inf$#  NSignals=12  IDPort=off  TimestampPort=off  ErrorPort=off  RemotePort=off  LengthPort=off  StatusPort=off  StartBits=str2num('[int32(54);int32(55);int32(24);int32(25);int32(36);int32(27);int32(26);int32(8);int32(16);int32(31);int32(32);int32(52)]')  SignalSizes=str2num('[int32(1);int32(1);int32(1);int32(1);int32(4);int32(4);int32(1);int32(16);int32(8);int32(1);int32(4);int32(2)]')  ByteOrders=str2num('[int32(2);int32(2);int32(2);int32(2);int32(2);int32(2);int32(2);int32(2);int32(2);int32(2);int32(2);int32(2)]')  DataTypes=str2num('[int32(2);int32(2);int32(2);int32(2);int32(2);int32(2);int32(2);int32(1);int32(2);int32(2);int32(2);int32(2)]')  MultiplexTypes=str2num('[int32(1);int32(1);int32(1);int32(1);int32(1);int32(1);int32(1);int32(1);int32(1);int32(1);int32(1);int32(1)]')  MultiplexValues=str2num('[double(0);double(0);double(0);double(0);double(0);double(0);double(0);double(0);double(0);double(0);double(0);double(0)]')  Factors=str2num('[double(1);double(1);double(1);double(1);double(1);double(1);double(1);double(1.000000e-01);double(4);double(1);double(1);double(1)]')  Offsets=str2num('[double(0);double(0);double(0);double(0);double(0);double(0);double(0);double(0);double(0);double(0);double(0);double(0)]')  Minimums=str2num('[double(-Inf);double(-Inf);double(-Inf);double(-Inf);double(-Inf);double(-Inf);double(-Inf);double(-780);double(0);double(-Inf);double(0);double(-Inf)]')  Maximums=str2num('[double(Inf);double(Inf);double(Inf);double(Inf);double(Inf);double(Inf);double(Inf);double(780);double(1016);double(Inf);double(15);double(Inf)]')  ApplyMinMax=off
      settings: SourceProductName=Simulink Real-Time  SourceProductBaseCode=XP  DataFormat=CANdb specified signals
  Data Type Conversion1 : DataTypeConversion  OutDataTypeStr=single
  Data Type Conversion2 : DataTypeConversion  OutDataTypeStr=single
  Data Type Conversion46 : DataTypeConversion  OutDataTypeStr=uint8
  Data Type Conversion47 : DataTypeConversion  OutDataTypeStr=uint8
  Rate Transition{1..12} (12 alike) : RateTransition  Deterministic=off  OutPortSampleTime=0.01
  Rate Transition13 : RateTransition  Deterministic=off  OutPortSampleTime=0.1
  Rate Transition14 : RateTransition  Deterministic=off  OutPortSampleTime=0.1
  Rate Transition15 : RateTransition  Deterministic=off  OutPortSampleTime=0.1
  Terminator{1..8} (8 alike) : Terminator
  bsSWAInfo : Outport
  wires:
  Data Type Conversion46/1 -> Bus Creator3/3  "SWS_Fault_Code"
  CAN Unpack1/4 -> Rate Transition7/1
  CAN Unpack1/5 -> Rate Transition8/1
  CAN Unpack1/11 -> Rate Transition10/1
  Bus Creator3/1 -> bsSWAInfo/1  "bsSWAInfo"
  CAN Unpack1/12 -> Rate Transition11/1
  CAN Unpack1/8 -> Rate Transition2/1  "SWARx_phiSWA"
  CAN Unpack1/2 -> Rate Transition6/1  "SWARx_phiSWA"
  CAN Unpack1/9 -> Rate Transition1/1  "SW_Angle_Speed"
  CAN Unpack1/10 -> Rate Transition12/1
  CAN Unpack1/6 -> Rate Transition4/1
  CAN Unpack1/3 -> Rate Transition3/1
  Data Type Conversion47/1 -> Bus Creator3/4  "SAS_In_Status"
  CAN Unpack1/1 -> Rate Transition5/1
  CAN Unpack1/7 -> Rate Transition9/1
  Data Type Conversion1/1 -> Rate Transition13/1, Bus Creator3/1  "SW_Angle"
  Data Type Conversion2/1 -> Rate Transition14/1, Bus Creator3/2  "SW_Angle_Speed"
  Rate Transition1/1 -> Data Type Conversion2/1
  Rate Transition2/1 -> Data Type Conversion1/1
  Rate Transition3/1 -> Data Type Conversion47/1
  Rate Transition4/1 -> Data Type Conversion46/1
  CAN Pack/1 -> CAN Send2/1
  Rate Transition5/1 -> Terminator1/1
  Rate Transition6/1 -> Terminator2/1
  Rate Transition7/1 -> Terminator3/1
  Rate Transition8/1 -> Terminator4/1
  Rate Transition9/1 -> Terminator5/1
  Rate Transition10/1 -> Terminator7/1
  Rate Transition11/1 -> Terminator8/1
  Rate Transition12/1 -> Rate Transition15/1, Terminator6/1
  Rate Transition13/1 -> CAN Pack/1
  Rate Transition14/1 -> CAN Pack/2
  Rate Transition15/1 -> CAN Pack/3
  CAN Recv (CANRx])/2 -> CAN Unpack1/1
